simulink model "w3_warplab_buffers"  (Simulink 7.7)
settings: Solver=VariableStepDiscrete  SolverMode=SingleTasking  StartTime=0.0  StopTime=200000  RelTol=1e-3
InitFcn:
  | w3_warplab_buffers_init
StartFcn:
  | w3_warplab_buffers_init
values from neighbouring files (symbols this model uses):
  NumSamps_Rx_IQ = 2^15    (= 32768)    [w3_warplab_buffers_init.m]
  NumSamps_Rx_RSSI = 2^13    (= 8192)    [w3_warplab_buffers_init.m]
  NumSamps_Tx_IQ = 2^15    (= 32768)    [w3_warplab_buffers_init.m]
undefined symbols (not defined in the file or in its folder): gcbh, xlBlockLoadCallback, xlGetNormalizedPeriod
libraries: xbsIndex_r4 x1266, xbsEDKLib_r4 x1
(part 3 of 9)

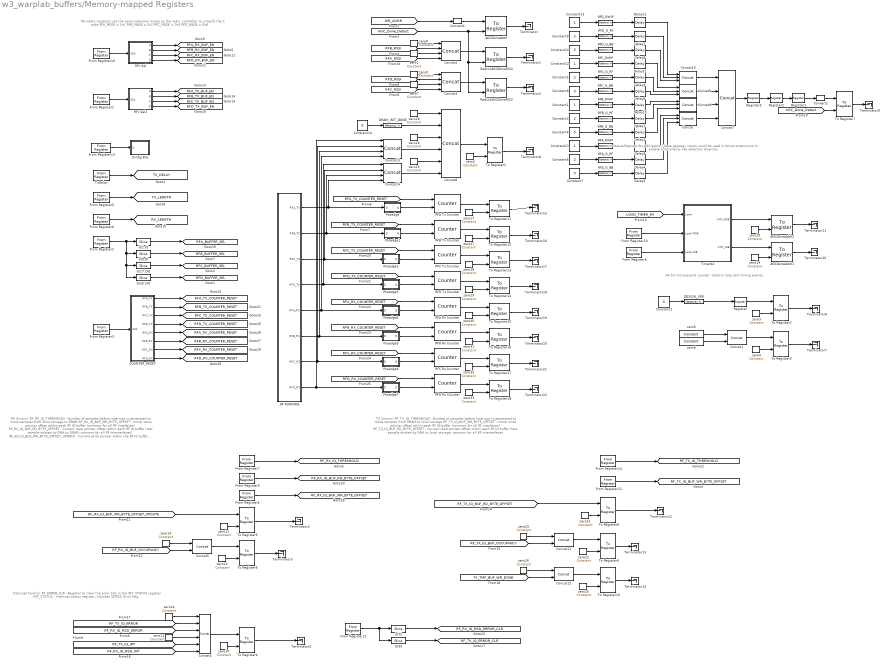
== system w3_warplab_buffers/Memory-mapped Registers ==
  note: Per-radio registers use the same selection
      | masks as the radio_controller to simplify the C code
      | RFA_MASK = 0x1
      | RFB_MASK = 0x2
      | RFC_MASK = 0x4
      | RFD_MASK = 0x8
  note: RX Control:
      |     RF_RX_IQ_THRESHOLD                                      - Number of samples before interrupt is generated to move samples from local storage to DRAM
      |     RF_RX_IQ_BUF_WR_BYTE_OFFSET                  - Initial write pointer offset within each RF IQ buffer (common for all RF interfaces)
      |     RF_RX_IQ_BUF_RD_BYTE_OFFSET                   - Current read pointer offset within each RF IQ buffer (last sample written by DMA to DRAM; common for all RF interterfaces)
      |     RF_RX_IQ_BUF_WR_BYTE_OFFSET_UPDATE  - Current write pointer within the RF IQ buffer (last sample written by RF interface; common for all RF interfaces)
  note: Status Register for AGC gains.  These gateway inputs could be used in future extensions to
      | enable functionality like selection diveristy.
  note: 64 bit microsecond counter. Used to help with timing events.
  note: TX Control:
      |     RF_TX_IQ_THRESHOLD                                      - Number of samples before interrupt is generated to move samples from DRAM to local storage
      |     RF_TX_IQ_BUF_WR_BYTE_OFFSET                  - Initial write pointer offset within each RF IQ buffer (common for all RF interfaces)
      |     RF_TX_IQ_BUF_RD_BYTE_OFFSET                   - Current read pointer offset within each RF IQ buffer (last sample written by DMA to local storage; common for all RF interterfaces
  note: Interrupt Control:
      |     RF_ERROR_CLR                                                   - Register to clear the error bits in the INT_STATUS register
      |     INT_STATUS                                                        - Interrupt status register; Includes IQ/RSSI Error flag
  AGCDoneAddr : xbsIndex_r4/To Register  shared_memory_name='AGC_DONE_ADDR'  init=0  ownership=Locally owned and initialized  explicit_data_type=on  gui_display_data_type=Fixed-point  arith_type=Unsigned  n_bits=32  bin_pt=0  preci_type=Single  dbl_ovrd=off  block_type=toreg
      settings: AttributesFormatString=<< %<shared_memory_name> >>  infoedit="Register block that writes data to a shared memory register.  Delay of one sample period."  block_version=10.1.3
  AGCDoneAddr1 : xbsIndex_r4/To Register  shared_memory_name='TIMER_64_LSB'  init=0  ownership=Locally owned and initialized  explicit_data_type=on  gui_display_data_type=Fixed-point  arith_type=Unsigned  n_bits=32  bin_pt=0  preci_type=Single  dbl_ovrd=off  block_type=toreg
      settings: AttributesFormatString=<< %<shared_memory_name> >>  infoedit="Register block that writes data to a shared memory register.  Delay of one sample period."  block_version=10.1.3
  AGCDoneAddr2 : xbsIndex_r4/To Register  shared_memory_name='TIMER_64_MSB'  init=0  ownership=Locally owned and initialized  explicit_data_type=on  gui_display_data_type=Fixed-point  arith_type=Unsigned  n_bits=32  bin_pt=0  preci_type=Single  dbl_ovrd=off  block_type=toreg
      settings: AttributesFormatString=<< %<shared_memory_name> >>  infoedit="Register block that writes data to a shared memory register.  Delay of one sample period."  block_version=10.1.3
  COUNTER_RESET : Subsystem
  Concat{,8..10} (4 alike) : xbsIndex_r4/Concat  num_inputs=3  dbl_ovrd=off  block_type=concat
  Concat{1,5,11..12} (4 alike) : xbsIndex_r4/Concat  num_inputs=2  dbl_ovrd=off  block_type=concat
  Concat{2..3,7,13..14} (5 alike) : xbsIndex_r4/Concat  num_inputs=4  dbl_ovrd=off  block_type=concat
  Concat4 : xbsIndex_r4/Concat  num_inputs=6  dbl_ovrd=off  block_type=concat
  Concat6 : xbsIndex_r4/Concat  num_inputs=6  dbl_ovrd=off  block_type=concat
  Config Bits : Subsystem
  Constant{1,11..13} (4 alike) : Constant
  Constant{4,7..8,10} (4 alike) : Constant  Value=5
  Constant14 : Constant  Value=0
  Constant2 : Constant  Value=0
  Constant{3,5..6,9} (4 alike) : Constant  Value=2
  Convert1 : xbsIndex_r4/Convert  gui_display_data_type=Fixed-point  arith_type=Unsigned  n_bits=32  bin_pt=0  float_type=Single  exp_bits=8  fraction_bits=24  quantization=Truncate  overflow=Wrap  en=off  latency=0  dbl_ovrd=off  pipeline=off  block_type=convert
      settings: block_version=8.2
  Convert4 : xbsIndex_r4/Convert  gui_display_data_type=Fixed-point  arith_type=Unsigned  n_bits=32  bin_pt=0  float_type=Single  exp_bits=8  fraction_bits=24  quantization=Truncate  overflow=Wrap  en=off  latency=0  dbl_ovrd=off  pipeline=off  block_type=convert
      settings: block_version=8.2
  DESIGN_VER : xbsIndex_r4/Gateway In  gui_display_data_type=Fixed-point  arith_type=Unsigned  n_bits=32  bin_pt=0  preci_type=Single  exp_width=8  frac_width=24  quantization="Round  (unbiased: +/- Inf)"  overflow=Saturate  period=1  dbl_ovrd=off  timing_constraint=None  locs_specified=off  LOCs={}  UseAsADC=off  ADCChannel='1'  inherit_from_input=off  hdl_port=on  block_type=gatewayin
      settings: block_version=VER_STRING_GOES_HERE
  DRAM_INIT_DONE : xbsIndex_r4/Gateway In  gui_display_data_type=Fixed-point  arith_type=Unsigned  n_bits=1  bin_pt=0  preci_type=Single  exp_width=8  frac_width=24  quantization="Round  (unbiased: +/- Inf)"  overflow=Saturate  period=1  dbl_ovrd=off  timing_constraint=None  locs_specified=off  LOCs={}  UseAsADC=off  ADCChannel='1'  inherit_from_input=off  hdl_port=on  block_type=gatewayin
      settings: block_version=VER_STRING_GOES_HERE
  Delay{1..12} (12 alike) : xbsIndex_r4/Delay  rst=off  infoeditControl=Selection of Reset will increase slice count due to use of real FFs and instead of SRLs  en=off  latency=1  dbl_ovrd=off  reg_retiming=off  block_type=delay
  From Register1 : xbsIndex_r4/From Register  shared_memory_name='TX_BUF_EN'  init=tx_buf_en  period=1  ownership=Locally owned and initialized  gui_display_data_type=Fixed-point  arith_type=Unsigned  n_bits=32  bin_pt=0  preci_type=Single  dbl_ovrd=off  block_type=fromreg
      settings: AttributesFormatString=<< %<shared_memory_name> >>  infoedit="Register block that reads data to a shared memory register.  Delay of one sample period."  block_version=8.2
  From Register10 : xbsIndex_r4/From Register  shared_memory_name='LOAD_TIMER_64_MSB'  init=0  period=1  ownership=Locally owned and initialized  gui_display_data_type=Fixed-point  arith_type=Unsigned  n_bits=32  bin_pt=0  preci_type=Single  dbl_ovrd=off  block_type=fromreg
      settings: AttributesFormatString=<< %<shared_memory_name> >>  infoedit="Register block that reads data to a shared memory register.  Delay of one sample period."  block_version=8.2
  From Register11 : xbsIndex_r4/From Register  shared_memory_name='RF_TX_IQ_BUF_WR_BYTE_OFFSET'  init=rf_tx_iq_buf_wr_byte_offset  period=1  ownership=Locally owned and initialized  gui_display_data_type=Fixed-point  arith_type=Unsigned  n_bits=32  bin_pt=0  preci_type=Single  dbl_ovrd=off  block_type=fromreg
      settings: AttributesFormatString=<< %<shared_memory_name> >>  infoedit="Register block that reads data to a shared memory register.  Delay of one sample period."  block_version=8.2
  From Register12 : xbsIndex_r4/From Register  shared_memory_name='RF_ERROR_CLR'  init=rf_error_clr  period=1  ownership=Locally owned and initialized  gui_display_data_type=Fixed-point  arith_type=Unsigned  n_bits=9  bin_pt=0  preci_type=Single  dbl_ovrd=off  block_type=fromreg
      settings: AttributesFormatString=<< %<shared_memory_name> >>  infoedit="Register block that reads data to a shared memory register.  Delay of one sample period."  block_version=8.2
  From Register13 : xbsIndex_r4/From Register  shared_memory_name='CONFIG'  init=wl_buffers_config_init  period=1  ownership=Locally owned and initialized  gui_display_data_type=Fixed-point  arith_type=Unsigned  n_bits=32  bin_pt=0  preci_type=Single  dbl_ovrd=off  block_type=fromreg
      settings: AttributesFormatString=<< %<shared_memory_name> >>  infoedit="Register block that reads data to a shared memory register.  Delay of one sample period."
  From Register14 : xbsIndex_r4/From Register  shared_memory_name='RF_TX_IQ_THRESHOLD'  init=rf_tx_iq_threshold  period=1  ownership=Locally owned and initialized  gui_display_data_type=Fixed-point  arith_type=Unsigned  n_bits=32  bin_pt=0  preci_type=Single  dbl_ovrd=off  block_type=fromreg
      settings: AttributesFormatString=<< %<shared_memory_name> >>  infoedit="Register block that reads data to a shared memory register.  Delay of one sample period."  block_version=8.2
  From Register16 : xbsIndex_r4/From Register  shared_memory_name='RX_BUF_EN'  init=rx_buf_en  period=1  ownership=Locally owned and initialized  gui_display_data_type=Fixed-point  arith_type=Unsigned  n_bits=32  bin_pt=0  preci_type=Single  dbl_ovrd=off  block_type=fromreg
      settings: AttributesFormatString=<< %<shared_memory_name> >>  infoedit="Register block that reads data to a shared memory register.  Delay of one sample period."  block_version=8.2
  From Register2 : xbsIndex_r4/From Register  shared_memory_name='RF_BUFFER_SEL'  init=wl_buffers_rf_buffer_sel  period=1  ownership=Locally owned and initialized  gui_display_data_type=Fixed-point  arith_type=Unsigned  n_bits=32  bin_pt=0  preci_type=Single  dbl_ovrd=off  block_type=fromreg
      settings: AttributesFormatString=<< %<shared_memory_name> >>  infoedit="Register block that reads data to a shared memory register.  Delay of one sample period."  block_version=8.2
  From Register3 : xbsIndex_r4/From Register  shared_memory_name='TXRX_COUNTER_RESET'  init=txrx_counter_reset  period=1  ownership=Locally owned and initialized  gui_display_data_type=Fixed-point  arith_type=Unsigned  n_bits=32  bin_pt=0  preci_type=Single  dbl_ovrd=off  block_type=fromreg
      settings: AttributesFormatString=<< %<shared_memory_name> >>  infoedit="Register block that reads data to a shared memory register.  Delay of one sample period."  block_version=8.2
  From Register4 : xbsIndex_r4/From Register  shared_memory_name='RF_RX_IQ_BUF_WR_BYTE_OFFSET'  init=rf_rx_iq_buf_wr_byte_offset  period=1  ownership=Locally owned and initialized  gui_display_data_type=Fixed-point  arith_type=Unsigned  n_bits=32  bin_pt=0  preci_type=Single  dbl_ovrd=off  block_type=fromreg
      settings: AttributesFormatString=<< %<shared_memory_name> >>  infoedit="Register block that reads data to a shared memory register.  Delay of one sample period."  block_version=8.2
  From Register5 : xbsIndex_r4/From Register  shared_memory_name='TX_LENGTH'  init=tx_length  period=1  ownership=Locally owned and initialized  gui_display_data_type=Fixed-point  arith_type=Unsigned  n_bits=32  bin_pt=0  preci_type=Single  dbl_ovrd=off  block_type=fromreg
      settings: AttributesFormatString=<< %<shared_memory_name> >>  infoedit="Register block that reads data to a shared memory register.  Delay of one sample period."  block_version=8.2
  From Register6 : xbsIndex_r4/From Register  shared_memory_name='RX_LENGTH'  init=rx_length  period=1  ownership=Locally owned and initialized  gui_display_data_type=Fixed-point  arith_type=Unsigned  n_bits=32  bin_pt=0  preci_type=Single  dbl_ovrd=off  block_type=fromreg
      settings: AttributesFormatString=<< %<shared_memory_name> >>  infoedit="Register block that reads data to a shared memory register.  Delay of one sample period."  block_version=8.2
  From Register7 : xbsIndex_r4/From Register  shared_memory_name='RF_RX_IQ_THRESHOLD'  init=rf_rx_iq_threshold  period=1  ownership=Locally owned and initialized  gui_display_data_type=Fixed-point  arith_type=Unsigned  n_bits=32  bin_pt=0  preci_type=Single  dbl_ovrd=off  block_type=fromreg
      settings: AttributesFormatString=<< %<shared_memory_name> >>  infoedit="Register block that reads data to a shared memory register.  Delay of one sample period."  block_version=8.2
  From Register8 : xbsIndex_r4/From Register  shared_memory_name='LOAD_TIMER_64_LSB'  init=0  period=1  ownership=Locally owned and initialized  gui_display_data_type=Fixed-point  arith_type=Unsigned  n_bits=32  bin_pt=0  preci_type=Single  dbl_ovrd=off  block_type=fromreg
      settings: AttributesFormatString=<< %<shared_memory_name> >>  infoedit="Register block that reads data to a shared memory register.  Delay of one sample period."  block_version=8.2
  From Register9 : xbsIndex_r4/From Register  shared_memory_name='RF_RX_IQ_BUF_RD_BYTE_OFFSET'  init=rf_rx_iq_buf_rd_byte_offset  period=1  ownership=Locally owned and initialized  gui_display_data_type=Fixed-point  arith_type=Unsigned  n_bits=32  bin_pt=0  preci_type=Single  dbl_ovrd=off  block_type=fromreg
      settings: AttributesFormatString=<< %<shared_memory_name> >>  infoedit="Register block that reads data to a shared memory register.  Delay of one sample period."  block_version=8.2
  Posedge : Subsystem
  Posedge1 : Subsystem
  Posedge2 : Subsystem
  Posedge3 : Subsystem
  Posedge4 : Subsystem
  Posedge5 : Subsystem
  Posedge6 : Subsystem
  Posedge7 : Subsystem
  RF RUNNING : Subsystem
  RFA Rx Counter : xbsIndex_r4/Counter  cnt_type=Free Running  cnt_to=Inf  operation=Up  start_count=0  cnt_by_val=1  arith_type=Unsigned  n_bits=32  bin_pt=0  load_pin=off  rst=on  en=on  explicit_period=off  period=1  dbl_ovrd=off  use_behavioral_HDL=off  implementation=Fabric  use_rpm=off  block_type=counter
      settings: block_version=8.2
  RFA Tx Counter : xbsIndex_r4/Counter  cnt_type=Free Running  cnt_to=Inf  operation=Up  start_count=0  cnt_by_val=1  arith_type=Unsigned  n_bits=32  bin_pt=0  load_pin=off  rst=on  en=on  explicit_period=off  period=1  dbl_ovrd=off  use_behavioral_HDL=off  implementation=Fabric  use_rpm=off  block_type=counter
      settings: block_version=8.2
  RFA_G_BB : xbsIndex_r4/Gateway In  gui_display_data_type=Fixed-point  arith_type=Unsigned  n_bits=5  bin_pt=0  preci_type=Single  exp_width=8  frac_width=24  quantization="Round  (unbiased: +/- Inf)"  overflow=Saturate  period=1  dbl_ovrd=off  timing_constraint=None  locs_specified=off  LOCs={}  UseAsADC=off  ADCChannel='1'  inherit_from_input=off  hdl_port=on  block_type=gatewayin
  RFA_G_RF : xbsIndex_r4/Gateway In  gui_display_data_type=Fixed-point  arith_type=Unsigned  n_bits=2  bin_pt=0  preci_type=Single  exp_width=8  frac_width=24  quantization="Round  (unbiased: +/- Inf)"  overflow=Saturate  period=1  dbl_ovrd=off  timing_constraint=None  locs_specified=off  LOCs={}  UseAsADC=off  ADCChannel='1'  inherit_from_input=off  hdl_port=on  block_type=gatewayin
  RFA_RXHP : xbsIndex_r4/Gateway In  gui_display_data_type=Fixed-point  arith_type=Unsigned  n_bits=1  bin_pt=0  preci_type=Single  exp_width=8  frac_width=24  quantization="Round  (unbiased: +/- Inf)"  overflow=Saturate  period=1  dbl_ovrd=off  timing_constraint=None  locs_specified=off  LOCs={}  UseAsADC=off  ADCChannel='1'  inherit_from_input=off  hdl_port=on  block_type=gatewayin
  RFB Rx Counter : xbsIndex_r4/Counter  cnt_type=Free Running  cnt_to=Inf  operation=Up  start_count=0  cnt_by_val=1  arith_type=Unsigned  n_bits=32  bin_pt=0  load_pin=off  rst=on  en=on  explicit_period=off  period=1  dbl_ovrd=off  use_behavioral_HDL=off  implementation=Fabric  use_rpm=off  block_type=counter
      settings: block_version=8.2
  RFB Tx Counter : xbsIndex_r4/Counter  cnt_type=Free Running  cnt_to=Inf  operation=Up  start_count=0  cnt_by_val=1  arith_type=Unsigned  n_bits=32  bin_pt=0  load_pin=off  rst=on  en=on  explicit_period=off  period=1  dbl_ovrd=off  use_behavioral_HDL=off  implementation=Fabric  use_rpm=off  block_type=counter
      settings: block_version=8.2
  RFB_G_BB : xbsIndex_r4/Gateway In  gui_display_data_type=Fixed-point  arith_type=Unsigned  n_bits=5  bin_pt=0  preci_type=Single  exp_width=8  frac_width=24  quantization="Round  (unbiased: +/- Inf)"  overflow=Saturate  period=1  dbl_ovrd=off  timing_constraint=None  locs_specified=off  LOCs={}  UseAsADC=off  ADCChannel='1'  inherit_from_input=off  hdl_port=on  block_type=gatewayin
  RFB_G_RF : xbsIndex_r4/Gateway In  gui_display_data_type=Fixed-point  arith_type=Unsigned  n_bits=2  bin_pt=0  preci_type=Single  exp_width=8  frac_width=24  quantization="Round  (unbiased: +/- Inf)"  overflow=Saturate  period=1  dbl_ovrd=off  timing_constraint=None  locs_specified=off  LOCs={}  UseAsADC=off  ADCChannel='1'  inherit_from_input=off  hdl_port=on  block_type=gatewayin
  RFB_RXHP : xbsIndex_r4/Gateway In  gui_display_data_type=Fixed-point  arith_type=Unsigned  n_bits=1  bin_pt=0  preci_type=Single  exp_width=8  frac_width=24  quantization="Round  (unbiased: +/- Inf)"  overflow=Saturate  period=1  dbl_ovrd=off  timing_constraint=None  locs_specified=off  LOCs={}  UseAsADC=off  ADCChannel='1'  inherit_from_input=off  hdl_port=on  block_type=gatewayin
  RFC Rx Counter : xbsIndex_r4/Counter  cnt_type=Free Running  cnt_to=Inf  operation=Up  start_count=0  cnt_by_val=1  arith_type=Unsigned  n_bits=32  bin_pt=0  load_pin=off  rst=on  en=on  explicit_period=off  period=1  dbl_ovrd=off  use_behavioral_HDL=off  implementation=Fabric  use_rpm=off  block_type=counter
      settings: block_version=8.2
  RFC Tx Counter : xbsIndex_r4/Counter  cnt_type=Free Running  cnt_to=Inf  operation=Up  start_count=0  cnt_by_val=1  arith_type=Unsigned  n_bits=32  bin_pt=0  load_pin=off  rst=on  en=on  explicit_period=off  period=1  dbl_ovrd=off  use_behavioral_HDL=off  implementation=Fabric  use_rpm=off  block_type=counter
      settings: block_version=8.2
  RFC_G_BB : xbsIndex_r4/Gateway In  gui_display_data_type=Fixed-point  arith_type=Unsigned  n_bits=5  bin_pt=0  preci_type=Single  exp_width=8  frac_width=24  quantization="Round  (unbiased: +/- Inf)"  overflow=Saturate  period=1  dbl_ovrd=off  timing_constraint=None  locs_specified=off  LOCs={}  UseAsADC=off  ADCChannel='1'  inherit_from_input=off  hdl_port=on  block_type=gatewayin
  RFC_G_RF : xbsIndex_r4/Gateway In  gui_display_data_type=Fixed-point  arith_type=Unsigned  n_bits=2  bin_pt=0  preci_type=Single  exp_width=8  frac_width=24  quantization="Round  (unbiased: +/- Inf)"  overflow=Saturate  period=1  dbl_ovrd=off  timing_constraint=None  locs_specified=off  LOCs={}  UseAsADC=off  ADCChannel='1'  inherit_from_input=off  hdl_port=on  block_type=gatewayin
  RFC_RXHP : xbsIndex_r4/Gateway In  gui_display_data_type=Fixed-point  arith_type=Unsigned  n_bits=1  bin_pt=0  preci_type=Single  exp_width=8  frac_width=24  quantization="Round  (unbiased: +/- Inf)"  overflow=Saturate  period=1  dbl_ovrd=off  timing_constraint=None  locs_specified=off  LOCs={}  UseAsADC=off  ADCChannel='1'  inherit_from_input=off  hdl_port=on  block_type=gatewayin
  RFD Rx Counter : xbsIndex_r4/Counter  cnt_type=Free Running  cnt_to=Inf  operation=Up  start_count=0  cnt_by_val=1  arith_type=Unsigned  n_bits=32  bin_pt=0  load_pin=off  rst=on  en=on  explicit_period=off  period=1  dbl_ovrd=off  use_behavioral_HDL=off  implementation=Fabric  use_rpm=off  block_type=counter
      settings: block_version=8.2
  RFD Tx Counter : xbsIndex_r4/Counter  cnt_type=Free Running  cnt_to=Inf  operation=Up  start_count=0  cnt_by_val=1  arith_type=Unsigned  n_bits=32  bin_pt=0  load_pin=off  rst=on  en=on  explicit_period=off  period=1  dbl_ovrd=off  use_behavioral_HDL=off  implementation=Fabric  use_rpm=off  block_type=counter
      settings: block_version=8.2
  RFD_G_BB : xbsIndex_r4/Gateway In  gui_display_data_type=Fixed-point  arith_type=Unsigned  n_bits=5  bin_pt=0  preci_type=Single  exp_width=8  frac_width=24  quantization="Round  (unbiased: +/- Inf)"  overflow=Saturate  period=1  dbl_ovrd=off  timing_constraint=None  locs_specified=off  LOCs={}  UseAsADC=off  ADCChannel='1'  inherit_from_input=off  hdl_port=on  block_type=gatewayin
  RFD_G_RF : xbsIndex_r4/Gateway In  gui_display_data_type=Fixed-point  arith_type=Unsigned  n_bits=2  bin_pt=0  preci_type=Single  exp_width=8  frac_width=24  quantization="Round  (unbiased: +/- Inf)"  overflow=Saturate  period=1  dbl_ovrd=off  timing_constraint=None  locs_specified=off  LOCs={}  UseAsADC=off  ADCChannel='1'  inherit_from_input=off  hdl_port=on  block_type=gatewayin
  RFD_RXHP : xbsIndex_r4/Gateway In  gui_display_data_type=Fixed-point  arith_type=Unsigned  n_bits=1  bin_pt=0  preci_type=Single  exp_width=8  frac_width=24  quantization="Round  (unbiased: +/- Inf)"  overflow=Saturate  period=1  dbl_ovrd=off  timing_constraint=None  locs_specified=off  LOCs={}  UseAsADC=off  ADCChannel='1'  inherit_from_input=off  hdl_port=on  block_type=gatewayin
  RFx Sel : Subsystem
  RFx Sel2 : Subsystem
  Radio1AGCDoneRSSI : xbsIndex_r4/To Register  shared_memory_name='RFAB_AGC_DONE_RSSI'  init=0  ownership=Locally owned and initialized  explicit_data_type=on  gui_display_data_type=Fixed-point  arith_type=Unsigned  n_bits=32  bin_pt=0  preci_type=Single  dbl_ovrd=off  block_type=toreg
      settings: AttributesFormatString=<< %<shared_memory_name> >>  infoedit="Register block that writes data to a shared memory register.  Delay of one sample period."  block_version=10.1.3
  Radio3AGCDoneRSSI : xbsIndex_r4/To Register  shared_memory_name='RFCD_AGC_DONE_RSSI'  init=0  ownership=Locally owned and initialized  explicit_data_type=on  gui_display_data_type=Fixed-point  arith_type=Unsigned  n_bits=32  bin_pt=0  preci_type=Single  dbl_ovrd=off  block_type=toreg
      settings: AttributesFormatString=<< %<shared_memory_name> >>  infoedit="Register block that writes data to a shared memory register.  Delay of one sample period."  block_version=10.1.3
  Register{,1..3} (4 alike) : xbsIndex_r4/Register  init=0  rst=off  en=off  dbl_ovrd=off  block_type=register
      settings: block_version=8.2
  Terminator{,1..22} (23 alike) : Terminator
  Timer64 : Subsystem
  To Register1 : xbsIndex_r4/To Register  shared_memory_name='STATUS'  init=0  ownership=Locally owned and initialized  explicit_data_type=on  gui_display_data_type=Fixed-point  arith_type=Unsigned  n_bits=32  bin_pt=0  preci_type=Single  dbl_ovrd=off  block_type=toreg
      settings: AttributesFormatString=<< %<shared_memory_name> >>  infoedit="Register block that writes data to a shared memory register.  Delay of one sample period."  block_version=8.2
  To Register10 : xbsIndex_r4/To Register  shared_memory_name='RF_TX_IQ_STATUS'  init=0  ownership=Locally owned and initialized  explicit_data_type=on  gui_display_data_type=Fixed-point  arith_type=Unsigned  n_bits=32  bin_pt=0  preci_type=Single  dbl_ovrd=off  block_type=toreg
      settings: AttributesFormatString=<< %<shared_memory_name> >>  infoedit="Register block that writes data to a shared memory register.  Delay of one sample period."  block_version=8.2
  To Register11 : xbsIndex_r4/To Register  shared_memory_name='RFA_TX_COUNTER'  init=0  ownership=Locally owned and initialized  explicit_data_type=on  gui_display_data_type=Fixed-point  arith_type=Unsigned  n_bits=32  bin_pt=0  preci_type=Single  dbl_ovrd=off  block_type=toreg
      settings: AttributesFormatString=<< %<shared_memory_name> >>  infoedit="Register block that writes data to a shared memory register.  Delay of one sample period."  block_version=8.2
  To Register12 : xbsIndex_r4/To Register  shared_memory_name='RFB_TX_COUNTER'  init=0  ownership=Locally owned and initialized  explicit_data_type=on  gui_display_data_type=Fixed-point  arith_type=Unsigned  n_bits=32  bin_pt=0  preci_type=Single  dbl_ovrd=off  block_type=toreg
      settings: AttributesFormatString=<< %<shared_memory_name> >>  infoedit="Register block that writes data to a shared memory register.  Delay of one sample period."  block_version=8.2
  To Register13 : xbsIndex_r4/To Register  shared_memory_name='RFC_TX_COUNTER'  init=0  ownership=Locally owned and initialized  explicit_data_type=on  gui_display_data_type=Fixed-point  arith_type=Unsigned  n_bits=32  bin_pt=0  preci_type=Single  dbl_ovrd=off  block_type=toreg
      settings: AttributesFormatString=<< %<shared_memory_name> >>  infoedit="Register block that writes data to a shared memory register.  Delay of one sample period."  block_version=8.2
  To Register14 : xbsIndex_r4/To Register  shared_memory_name='RFD_TX_COUNTER'  init=0  ownership=Locally owned and initialized  explicit_data_type=on  gui_display_data_type=Fixed-point  arith_type=Unsigned  n_bits=32  bin_pt=0  preci_type=Single  dbl_ovrd=off  block_type=toreg
      settings: AttributesFormatString=<< %<shared_memory_name> >>  infoedit="Register block that writes data to a shared memory register.  Delay of one sample period."  block_version=8.2
  To Register15 : xbsIndex_r4/To Register  shared_memory_name='RFA_RX_COUNTER'  init=0  ownership=Locally owned and initialized  explicit_data_type=on  gui_display_data_type=Fixed-point  arith_type=Unsigned  n_bits=32  bin_pt=0  preci_type=Single  dbl_ovrd=off  block_type=toreg
      settings: AttributesFormatString=<< %<shared_memory_name> >>  infoedit="Register block that writes data to a shared memory register.  Delay of one sample period."  block_version=8.2
  To Register16 : xbsIndex_r4/To Register  shared_memory_name='RFB_RX_COUNTER'  init=0  ownership=Locally owned and initialized  explicit_data_type=on  gui_display_data_type=Fixed-point  arith_type=Unsigned  n_bits=32  bin_pt=0  preci_type=Single  dbl_ovrd=off  block_type=toreg
      settings: AttributesFormatString=<< %<shared_memory_name> >>  infoedit="Register block that writes data to a shared memory register.  Delay of one sample period."  block_version=8.2
  To Register17 : xbsIndex_r4/To Register  shared_memory_name='RFC_RX_COUNTER'  init=0  ownership=Locally owned and initialized  explicit_data_type=on  gui_display_data_type=Fixed-point  arith_type=Unsigned  n_bits=32  bin_pt=0  preci_type=Single  dbl_ovrd=off  block_type=toreg
      settings: AttributesFormatString=<< %<shared_memory_name> >>  infoedit="Register block that writes data to a shared memory register.  Delay of one sample period."  block_version=8.2
  To Register18 : xbsIndex_r4/To Register  shared_memory_name='RFD_RX_COUNTER'  init=0  ownership=Locally owned and initialized  explicit_data_type=on  gui_display_data_type=Fixed-point  arith_type=Unsigned  n_bits=32  bin_pt=0  preci_type=Single  dbl_ovrd=off  block_type=toreg
      settings: AttributesFormatString=<< %<shared_memory_name> >>  infoedit="Register block that writes data to a shared memory register.  Delay of one sample period."  block_version=8.2
  To Register2 : xbsIndex_r4/To Register  shared_memory_name='DESIGN_VER'  init=0  ownership=Locally owned and initialized  explicit_data_type=on  gui_display_data_type=Fixed-point  arith_type=Unsigned  n_bits=32  bin_pt=0  preci_type=Single  dbl_ovrd=off  block_type=toreg
      settings: AttributesFormatString=<< %<shared_memory_name> >>  infoedit="Register block that writes data to a shared memory register.  Delay of one sample period."  block_version=8.2
  To Register3 : xbsIndex_r4/To Register  shared_memory_name='BUFF_SIZES'  init=0  ownership=Locally owned and initialized  explicit_data_type=on  gui_display_data_type=Fixed-point  arith_type=Unsigned  n_bits=32  bin_pt=0  preci_type=Single  dbl_ovrd=off  block_type=toreg
      settings: AttributesFormatString=<< %<shared_memory_name> >>  infoedit="Register block that writes data to a shared memory register.  Delay of one sample period."  block_version=8.2
  To Register4 : xbsIndex_r4/To Register  shared_memory_name='INT_STATUS'  init=0  ownership=Locally owned and initialized  explicit_data_type=on  gui_display_data_type=Fixed-point  arith_type=Unsigned  n_bits=32  bin_pt=0  preci_type=Single  dbl_ovrd=off  block_type=toreg
      settings: AttributesFormatString=<< %<shared_memory_name> >>  infoedit="Register block that writes data to a shared memory register.  Delay of one sample period."  block_version=8.2
  To Register5 : xbsIndex_r4/To Register  shared_memory_name='RF_RX_IQ_BUF_WR_BYTE_OFFSET_UPDATE'  init=0  ownership=Locally owned and initialized  explicit_data_type=on  gui_display_data_type=Fixed-point  arith_type=Unsigned  n_bits=32  bin_pt=0  preci_type=Single  dbl_ovrd=off  block_type=toreg
      settings: AttributesFormatString=<< %<shared_memory_name> >>  infoedit="Register block that writes data to a shared memory register.  Delay of one sample period."  block_version=8.2
  To Register6 : xbsIndex_r4/To Register  shared_memory_name='RF_RX_IQ_BUF_OCCUPANCY'  init=0  ownership=Locally owned and initialized  explicit_data_type=on  gui_display_data_type=Fixed-point  arith_type=Unsigned  n_bits=32  bin_pt=0  preci_type=Single  dbl_ovrd=off  block_type=toreg
      settings: AttributesFormatString=<< %<shared_memory_name> >>  infoedit="Register block that writes data to a shared memory register.  Delay of one sample period."  block_version=8.2
  To Register7 : xbsIndex_r4/To Register  shared_memory_name='AGC_GAINS'  init=0  ownership=Locally owned and initialized  explicit_data_type=on  gui_display_data_type=Fixed-point  arith_type=Unsigned  n_bits=32  bin_pt=0  preci_type=Single  dbl_ovrd=off  block_type=toreg
      settings: AttributesFormatString=<< %<shared_memory_name> >>  infoedit="Register block that writes data to a shared memory register.  Delay of one sample period."  block_version=8.2
  To Register8 : xbsIndex_r4/To Register  shared_memory_name='RF_TX_IQ_BUF_RD_BYTE_OFFSET'  init=0  ownership=Locally owned and initialized  explicit_data_type=on  gui_display_data_type=Fixed-point  arith_type=Unsigned  n_bits=32  bin_pt=0  preci_type=Single  dbl_ovrd=off  block_type=toreg
      settings: AttributesFormatString=<< %<shared_memory_name> >>  infoedit="Register block that writes data to a shared memory register.  Delay of one sample period."  block_version=8.2
  To Register9 : xbsIndex_r4/To Register  shared_memory_name='RF_TX_IQ_BUF_OCCUPANCY'  init=0  ownership=Locally owned and initialized  explicit_data_type=on  gui_display_data_type=Fixed-point  arith_type=Unsigned  n_bits=32  bin_pt=0  preci_type=Single  dbl_ovrd=off  block_type=toreg
      settings: AttributesFormatString=<< %<shared_memory_name> >>  infoedit="Register block that writes data to a shared memory register.  Delay of one sample period."  block_version=8.2
  TxDelay : xbsIndex_r4/From Register  shared_memory_name='TX_DELAY'  init=wl_buffers_tx_delay_init  period=1  ownership=Locally owned and initialized  gui_display_data_type=Fixed-point  arith_type=Unsigned  n_bits=32  bin_pt=0  preci_type=Single  dbl_ovrd=off  block_type=fromreg
      settings: AttributesFormatString=<< %<shared_memory_name> >>  infoedit="Register block that reads data to a shared memory register.  Delay of one sample period."  block_version=10.1.2
  b[0] : xbsIndex_r4/Slice  nbits=1  boolean_output=off  mode=Lower Bit Location + Width  bit1=0  base1=MSB of Input  bit0=0  base0=LSB of Input  dbl_ovrd=off  block_type=slice
  b[17:16] : xbsIndex_r4/Slice  nbits=2  boolean_output=off  mode=Lower Bit Location + Width  bit1=0  base1=MSB of Input  bit0=16  base0=LSB of Input  dbl_ovrd=off  block_type=slice
  b[1:0] : xbsIndex_r4/Slice  nbits=2  boolean_output=off  mode=Lower Bit Location + Width  bit1=0  base1=MSB of Input  bit0=0  base0=LSB of Input  dbl_ovrd=off  block_type=slice
  b[25:24] : xbsIndex_r4/Slice  nbits=2  boolean_output=off  mode=Lower Bit Location + Width  bit1=0  base1=MSB of Input  bit0=24  base0=LSB of Input  dbl_ovrd=off  block_type=slice
  b[8] : xbsIndex_r4/Slice  nbits=1  boolean_output=off  mode=Lower Bit Location + Width  bit1=0  base1=MSB of Input  bit0=8  base0=LSB of Input  dbl_ovrd=off  block_type=slice
  b[9:8] : xbsIndex_r4/Slice  nbits=2  boolean_output=off  mode=Lower Bit Location + Width  bit1=0  base1=MSB of Input  bit0=8  base0=LSB of Input  dbl_ovrd=off  block_type=slice
  zero{1,7..9,24} (5 alike) : xbsIndex_r4/Constant  const=0  gui_display_data_type=Fixed-point  arith_type=Unsigned  n_bits=6  bin_pt=0  preci_type=Single  exp_width=8  frac_width=24  explicit_period=off  period=1  equ=P=C  opselect=C  inp2=PCIN>>17  opr=+  inp1=P  carry=CIN  dbl_ovrd=off  block_type=constant
      settings: block_version=VER_STRING_GOES_HERE
  zero{2..4,10,12..13,17,19..22,25,27..33} (19 alike) : xbsIndex_r4/Constant  const=1  gui_display_data_type=Fixed-point  arith_type=Boolean  n_bits=1  bin_pt=0  preci_type=Single  exp_width=8  frac_width=24  explicit_period=off  period=1  equ=P=C  opselect=C  inp2=PCIN>>17  opr=+  inp1=P  carry=CIN  dbl_ovrd=off  block_type=constant
      settings: block_version=VER_STRING_GOES_HERE
  zero11 : xbsIndex_r4/Constant  const=0  gui_display_data_type=Fixed-point  arith_type=Unsigned  n_bits=22  bin_pt=0  preci_type=Single  exp_width=8  frac_width=24  explicit_period=off  period=1  equ=P=C  opselect=C  inp2=PCIN>>17  opr=+  inp1=P  carry=CIN  dbl_ovrd=off  block_type=constant
      settings: block_version=VER_STRING_GOES_HERE
  zero14 : xbsIndex_r4/Constant  const=0  gui_display_data_type=Fixed-point  arith_type=Unsigned  n_bits=2  bin_pt=0  preci_type=Single  exp_width=8  frac_width=24  explicit_period=off  period=1  equ=P=C  opselect=C  inp2=PCIN>>17  opr=+  inp1=P  carry=CIN  dbl_ovrd=off  block_type=constant
      settings: block_version=VER_STRING_GOES_HERE
  zero15 : xbsIndex_r4/Constant  const=0  gui_display_data_type=Fixed-point  arith_type=Unsigned  n_bits=4  bin_pt=0  preci_type=Single  exp_width=8  frac_width=24  explicit_period=off  period=1  equ=P=C  opselect=C  inp2=PCIN>>17  opr=+  inp1=P  carry=CIN  dbl_ovrd=off  block_type=constant
      settings: block_version=VER_STRING_GOES_HERE
  zero16 : xbsIndex_r4/Constant  const=0  gui_display_data_type=Fixed-point  arith_type=Unsigned  n_bits=4  bin_pt=0  preci_type=Single  exp_width=8  frac_width=24  explicit_period=off  period=1  equ=P=C  opselect=C  inp2=PCIN>>17  opr=+  inp1=P  carry=CIN  dbl_ovrd=off  block_type=constant
      settings: block_version=VER_STRING_GOES_HERE
  zero18 : xbsIndex_r4/Constant  const=0  gui_display_data_type=Fixed-point  arith_type=Unsigned  n_bits=15  bin_pt=0  preci_type=Single  exp_width=8  frac_width=24  explicit_period=off  period=1  equ=P=C  opselect=C  inp2=PCIN>>17  opr=+  inp1=P  carry=CIN  dbl_ovrd=off  block_type=constant
      settings: block_version=VER_STRING_GOES_HERE
  zero23 : xbsIndex_r4/Constant  const=0  gui_display_data_type=Fixed-point  arith_type=Unsigned  n_bits=2  bin_pt=0  preci_type=Single  exp_width=8  frac_width=24  explicit_period=off  period=1  equ=P=C  opselect=C  inp2=PCIN>>17  opr=+  inp1=P  carry=CIN  dbl_ovrd=off  block_type=constant
      settings: block_version=VER_STRING_GOES_HERE
  zero26 : xbsIndex_r4/Constant  const=0  gui_display_data_type=Fixed-point  arith_type=Unsigned  n_bits=31  bin_pt=0  preci_type=Single  exp_width=8  frac_width=24  explicit_period=off  period=1  equ=P=C  opselect=C  inp2=PCIN>>17  opr=+  inp1=P  carry=CIN  dbl_ovrd=off  block_type=constant
      settings: block_version=VER_STRING_GOES_HERE
  zero5 : xbsIndex_r4/Constant  const=NumSamps_Tx_IQ  gui_display_data_type=Fixed-point  arith_type=Unsigned  n_bits=16  bin_pt=0  preci_type=Single  exp_width=8  frac_width=24  explicit_period=on  period=1  equ=P=C  opselect=C  inp2=PCIN>>17  opr=+  inp1=P  carry=CIN  dbl_ovrd=off  block_type=constant
      settings: block_version=VER_STRING_GOES_HERE
  zero6 : xbsIndex_r4/Constant  const=NumSamps_Rx_IQ  gui_display_data_type=Fixed-point  arith_type=Unsigned  n_bits=16  bin_pt=0  preci_type=Single  exp_width=8  frac_width=24  explicit_period=on  period=1  equ=P=C  opselect=C  inp2=PCIN>>17  opr=+  inp1=P  carry=CIN  dbl_ovrd=off  block_type=constant
      settings: block_version=VER_STRING_GOES_HERE
  tag scope: RFA_BUFFER_SEL=global, RFA_RX_BUF_EN=global, RFA_RX_COUNTER_RESET=global, RFA_TX_BUF_EN=global, RFA_TX_COUNTER_RESET=global, RFB_BUFFER_SEL=global, RFB_RX_BUF_EN=global, RFB_RX_COUNTER_RESET=global, RFB_TX_BUF_EN=global, RFB_TX_COUNTER_RESET=global, RFC_BUFFER_SEL=global, RFC_RX_BUF_EN=global, RFC_RX_COUNTER_RESET=global, RFC_TX_BUF_EN=global, RFC_TX_COUNTER_RESET=global, RFD_BUFFER_SEL=global, RFD_RX_BUF_EN=global, RFD_RX_COUNTER_RESET=global, RFD_TX_BUF_EN=global, RFD_TX_COUNTER_RESET=global, RF_RX_IQ_BUF_RD_BYTE_OFFSET=global, RF_RX_IQ_BUF_WR_BYTE_OFFSET=global, RF_RX_IQ_RSSI_ERROR_CLR=global, RF_RX_IQ_THRESHOLD=global, RF_TX_IQ_BUF_WR_BYTE_OFFSET=global, RF_TX_IQ_ERROR_CLR=global, RF_TX_IQ_THRESHOLD=global, RX_LENGTH=global, TX_DELAY=global, TX_LENGTH=global
  wires:
  TxDelay/1 -> [TX_DELAY]
  [AGC_Done_Detect] -> AGCDoneAddr/2, Radio1AGCDoneRSSI/2, Radio3AGCDoneRSSI/2
  Convert4/1 -> AGCDoneAddr/1
  Concat3/1 -> Radio3AGCDoneRSSI/1
  Concat2/1 -> Radio1AGCDoneRSSI/1
  From Register16/1 -> RFx Sel/1(32b)
  RFx Sel/1(A) -> [RFA_RX_BUF_EN]
  RFx Sel/2(B) -> [RFB_RX_BUF_EN]
  RFx Sel/3(C) -> [RFC_RX_BUF_EN]
  RFx Sel/4(D) -> [RFD_RX_BUF_EN]
  From Register1/1 -> RFx Sel2/1(32b)
  RFx Sel2/1(A) -> [RFA_TX_BUF_EN]
  RFx Sel2/2(B) -> [RFB_TX_BUF_EN]
  RFx Sel2/3(C) -> [RFC_TX_BUF_EN]
  RFx Sel2/4(D) -> [RFD_TX_BUF_EN]
  AGCDoneAddr/1 -> Terminator/1
  Radio1AGCDoneRSSI/1 -> Terminator1/1
  Radio3AGCDoneRSSI/1 -> Terminator3/1
  zero2/1 -> To Register1/2
  To Register1/1 -> Terminator6/1
  DESIGN_VER/1 -> Register/1
  zero3/1 -> To Register2/2
  Register/1 -> To Register2/1
  zero4/1 -> To Register3/2
  Concat1/1 -> To Register3/1
  zero5/1 -> Concat1/1
  zero6/1 -> Concat1/2
  To Register3/1 -> Terminator7/1
  To Register2/1 -> Terminator8/1
  From Register5/1 -> [TX_LENGTH]
  [WR_ADDR] -> Convert4/1
  From Register6/1 -> [RX_LENGTH]
  From Register13/1 -> Config Bits/1(D)
  zero1/1 -> Concat2/3
  [RFA_RSSI] -> Concat2/4
  [RFB_RSSI] -> Concat2/2
  zero8/1 -> Concat2/1
  zero7/1 -> Concat3/3
  [RFC_RSSI] -> Concat3/4
  zero9/1 -> Concat3/1
  [RFD_RSSI] -> Concat3/2
  b[1:0]/1 -> [RFA_BUFFER_SEL]
  b[9:8]/1 -> [RFB_BUFFER_SEL]
  b[17:16]/1 -> [RFC_BUFFER_SEL]
  b[25:24]/1 -> [RFD_BUFFER_SEL]
  From Register2/1 -> b[1:0]/1, b[9:8]/1, b[17:16]/1, b[25:24]/1
  From Register7/1 -> [RF_RX_IQ_THRESHOLD]
  From Register9/1 -> [RF_RX_IQ_BUF_RD_BYTE_OFFSET]
  Concat4/1 -> To Register4/1
  zero10/1 -> To Register4/2
  [RF_RX_IQ_BUF_WR_BYTE_OFFSET_UPDATE] -> To Register5/1
  To Register4/1 -> Terminator2/1
  From Register4/1 -> [RF_RX_IQ_BUF_WR_BYTE_OFFSET]
  To Register5/1 -> Terminator4/1
  zero12/1 -> To Register5/2
  zero13/1 -> To Register6/2
  Concat5/1 -> To Register6/1
  To Register6/1 -> Terminator5/1
  [RF_RX_IQ_BUF_OCCUPANCY] -> Concat5/2
  zero14/1 -> Concat5/1
  Constant2/1 -> DESIGN_VER/1
  Concat6/1 -> To Register1/1
  RFA_G_RF/1 -> Delay4/1
  RFA_G_BB/1 -> Delay5/1
  Constant6/1 -> RFA_G_RF/1
  Constant7/1 -> RFA_G_BB/1
  RFB_G_RF/1 -> Delay1/1
  RFB_G_BB/1 -> Delay2/1
  Constant3/1 -> RFB_G_RF/1
  Constant4/1 -> RFB_G_BB/1
  RFC_G_RF/1 -> Delay3/1
  RFC_G_BB/1 -> Delay6/1
  Constant5/1 -> RFC_G_RF/1
  Constant8/1 -> RFC_G_BB/1
  RFD_G_RF/1 -> Delay7/1
  RFD_G_BB/1 -> Delay8/1
  Constant9/1 -> RFD_G_RF/1
  Constant10/1 -> RFD_G_BB/1
  [AGC_Done_Detect] -> To Register7/2
  To Register7/1 -> Terminator9/1
  Concat7/1 -> Register3/1
  Register3/1 -> Register2/1
  Register2/1 -> Register1/1
  Register1/1 -> Convert1/1
  Convert1/1 -> To Register7/1
  RFA_RXHP/1 -> Delay9/1
  Constant11/1 -> RFA_RXHP/1
  RFB_RXHP/1 -> Delay10/1
  Constant1/1 -> RFB_RXHP/1
  RFC_RXHP/1 -> Delay11/1
  Constant12/1 -> RFC_RXHP/1
  RFD_RXHP/1 -> Delay12/1
  Constant13/1 -> RFD_RXHP/1
  Concat10/1 -> Concat7/1
  Concat9/1 -> Concat7/2
  Concat8/1 -> Concat7/3
  Concat/1 -> Concat7/4
  Delay12/1 -> Concat10/1
  Delay7/1 -> Concat10/2
  Delay8/1 -> Concat10/3
  Delay11/1 -> Concat9/1
  Delay3/1 -> Concat9/2
  Delay6/1 -> Concat9/3
  Delay10/1 -> Concat8/1
  Delay1/1 -> Concat8/2
  Delay2/1 -> Concat8/3
  Delay9/1 -> Concat/1
  Delay4/1 -> Concat/2
  Delay5/1 -> Concat/3
  AGCDoneAddr1/1 -> Terminator10/1
  Constant14/1 -> DRAM_INIT_DONE/1
  zero18/1 -> Concat6/1
  DRAM_INIT_DONE/1 -> Concat6/2
  zero19/1 -> AGCDoneAddr1/2
  AGCDoneAddr2/1 -> Terminator11/1
  zero20/1 -> AGCDoneAddr2/2
  From Register10/1 -> Timer64/2(Load MSB)
  From Register8/1 -> Timer64/3(Load LSB)
  Timer64/1(CNT_MSB) -> AGCDoneAddr2/1
  Timer64/2(CNT_LSB) -> AGCDoneAddr1/1
  [LOAD_TIMER_64] -> Timer64/1(Load)
  From Register14/1 -> [RF_TX_IQ_THRESHOLD]
  From Register11/1 -> [RF_TX_IQ_BUF_WR_BYTE_OFFSET]
  [RF_TX_IQ_BUF_RD_BYTE_OFFSET] -> To Register8/1
  To Register8/1 -> Terminator12/1
  zero21/1 -> To Register8/2
  zero22/1 -> To Register9/2
  Concat11/1 -> To Register9/1
  To Register9/1 -> Terminator13/1
  [RF_TX_IQ_BUF_OCCUPANCY] -> Concat11/2
  zero23/1 -> Concat11/1
  b[0]/1 -> [RF_RX_IQ_RSSI_ERROR_CLR]
  b[8]/1 -> [RF_TX_IQ_ERROR_CLR]
  From Register12/1 -> b[0]/1, b[8]/1
  zero11/1 -> Concat4/4
  [RF_TX_IQ_INT] -> Concat4/5
  [RF_RX_IQ_RSSI_INT] -> Concat4/6
  zero24/1 -> Concat4/1
  [RF_TX_IQ_ERROR] -> Concat4/2
  [RF_RX_IQ_RSSI_ERROR] -> Concat4/3
  zero25/1 -> To Register10/2
  Concat12/1 -> To Register10/1
  To Register10/1 -> Terminator14/1
  [TX_TMP_BUF_WR_DONE] -> Concat12/2
  zero26/1 -> Concat12/1
  zero16/1 -> Concat6/3
  Concat13/1 -> Concat6/4
  zero15/1 -> Concat6/5
  Concat14/1 -> Concat6/6
  zero17/1 -> To Register11/2
  RFA Tx Counter/1 -> To Register11/1
  To Register11/1 -> Terminator15/1
  zero27/1 -> To Register12/2
  RFB Tx Counter/1 -> To Register12/1
  To Register12/1 -> Terminator16/1
  zero28/1 -> To Register13/2
  RFC Tx Counter/1 -> To Register13/1
  To Register13/1 -> Terminator17/1
  zero29/1 -> To Register14/2
  RFD Tx Counter/1 -> To Register14/1
  To Register14/1 -> Terminator18/1
  zero30/1 -> To Register15/2
  RFA Rx Counter/1 -> To Register15/1
  To Register15/1 -> Terminator19/1
  zero31/1 -> To Register16/2
  RFB Rx Counter/1 -> To Register16/1
  To Register16/1 -> Terminator20/1
  zero32/1 -> To Register17/2
  RFC Rx Counter/1 -> To Register17/1
  To Register17/1 -> Terminator21/1
  zero33/1 -> To Register18/2
  RFD Rx Counter/1 -> To Register18/1
  To Register18/1 -> Terminator22/1
  COUNTER_RESET/1(RFA_TX) -> [RFA_TX_COUNTER_RESET]
  COUNTER_RESET/2(RFB_TX) -> [RFB_TX_COUNTER_RESET]
  COUNTER_RESET/3(RFC_TX) -> [RFC_TX_COUNTER_RESET]
  COUNTER_RESET/4(RFD_TX) -> [RFD_TX_COUNTER_RESET]
  COUNTER_RESET/5(RFA_RX) -> [RFA_RX_COUNTER_RESET]
  COUNTER_RESET/6(RFB_RX) -> [RFB_RX_COUNTER_RESET]
  COUNTER_RESET/7(RFC_RX) -> [RFC_RX_COUNTER_RESET]
  COUNTER_RESET/8(RFD_RX) -> [RFD_RX_COUNTER_RESET]
  From Register3/1 -> COUNTER_RESET/1(32b)
  [RFA_TX_COUNTER_RESET] -> RFA Tx Counter/1
  Posedge/1(Q) -> RFA Tx Counter/2
  [RFB_TX_COUNTER_RESET] -> RFB Tx Counter/1
  Posedge1/1(Q) -> RFB Tx Counter/2
  [RFC_TX_COUNTER_RESET] -> RFC Tx Counter/1
  Posedge2/1(Q) -> RFC Tx Counter/2
  [RFD_TX_COUNTER_RESET] -> RFD Tx Counter/1
  Posedge3/1(Q) -> RFD Tx Counter/2
  [RFA_RX_COUNTER_RESET] -> RFA Rx Counter/1
  Posedge4/1(Q) -> RFA Rx Counter/2
  [RFB_RX_COUNTER_RESET] -> RFB Rx Counter/1
  Posedge5/1(Q) -> RFB Rx Counter/2
  [RFC_RX_COUNTER_RESET] -> RFC Rx Counter/1
  Posedge6/1(Q) -> RFC Rx Counter/2
  [RFD_RX_COUNTER_RESET] -> RFD Rx Counter/1
  Posedge7/1(Q) -> RFD Rx Counter/2
  RF RUNNING/1(RFA_TX) -> Posedge/1(D), Concat14/4
  RF RUNNING/2(RFB_TX) -> Posedge1/1(D), Concat14/3
  RF RUNNING/3(RFC_TX) -> Posedge2/1(D), Concat14/2
  RF RUNNING/4(RFD_TX) -> Posedge3/1(D), Concat14/1
  RF RUNNING/5(RFA_RX) -> Posedge4/1(D), Concat13/4
  RF RUNNING/6(RFB_RX) -> Posedge5/1(D), Concat13/3
  RF RUNNING/7(RFC_RX) -> Posedge6/1(D), Concat13/2
  RF RUNNING/8(RFD_RX) -> Posedge7/1(D), Concat13/1

== system w3_warplab_buffers/Posedge 0 ==
  D : Inport
  Delay : xbsIndex_r4/Delay  rst=off  infoeditControl=Selection of Reset will increase slice count due to use of real FFs and instead of SRLs  en=off  latency=1  dbl_ovrd=off  reg_retiming=off  block_type=delay
      settings: infoedit=Hardware notes: A delay line is a chain, each link of which is an SRL16 followed by a flip-flop. If register retiming is enabled, the delay line is a chain of flip-flops.  block_version=8.2
  Inverter : xbsIndex_r4/Inverter  en=off  latency=0  dbl_ovrd=off  block_type=inv
      settings: block_version=8.2
  Logical : xbsIndex_r4/Logical  logical_function=AND  inputs=2  en=off  latency=0  precision=Full  arith_type=Unsigned  n_bits=16  bin_pt=0  align_bp=on  dbl_ovrd=off  block_type=logical
      settings: block_version=8.2
  Q : Outport
  wires:
  Logical/1 -> Q/1
  Delay/1 -> Logical/2
  Inverter/1 -> Delay/1
  D/1 -> Logical/1, Inverter/1

== system w3_warplab_buffers/Posedge 1 ==
  D : Inport
  Delay : xbsIndex_r4/Delay  rst=off  infoeditControl=Selection of Reset will increase slice count due to use of real FFs and instead of SRLs  en=off  latency=1  dbl_ovrd=off  reg_retiming=off  block_type=delay
      settings: infoedit=Hardware notes: A delay line is a chain, each link of which is an SRL16 followed by a flip-flop. If register retiming is enabled, the delay line is a chain of flip-flops.  block_version=8.2
  Inverter : xbsIndex_r4/Inverter  en=off  latency=0  dbl_ovrd=off  block_type=inv
      settings: block_version=8.2
  Logical : xbsIndex_r4/Logical  logical_function=AND  inputs=2  en=off  latency=0  precision=Full  arith_type=Unsigned  n_bits=16  bin_pt=0  align_bp=on  dbl_ovrd=off  block_type=logical
      settings: block_version=8.2
  Q : Outport
  wires:
  D/1 -> Inverter/1, Logical/1
  Inverter/1 -> Delay/1
  Delay/1 -> Logical/2
  Logical/1 -> Q/1

== system w3_warplab_buffers/RFA Rx Buffers ==
  RSSI : Inport
  I/Q : Inport  Port=2
  Addr : Inport  Port=3
  WE : Inport  Port=4
  EN : Inport  Port=5
  Convert1 : xbsIndex_r4/Convert  gui_display_data_type=Fixed-point  arith_type=Boolean  n_bits=16  bin_pt=14  float_type=Single  exp_bits=8  fraction_bits=24  quantization=Truncate  overflow=Wrap  en=off  latency=0  dbl_ovrd=off  pipeline=off  block_type=convert
      settings: block_version=8.2
  Gateway Out : xbsIndex_r4/Gateway Out  inherit_from_input=off  hdl_port=off  timing_constraint=None  locs_specified=off  LOCs={}  UseAsDAC=off  DACChannel='1'  block_type=gatewayout
      settings: infoedit="Gateway out block.  Converts Xilinx fixed point inputs into ouputs of type Simulink integer, double, or fixed point.<P><P>Hardware notes:  In hardware these blocks become top level output ports or are discarded, depending on how they are configured."  block_version=10.1.2
  Gateway Out1 : xbsIndex_r4/Gateway Out  inherit_from_input=off  hdl_port=off  timing_constraint=None  locs_specified=off  LOCs={}  UseAsDAC=off  DACChannel='1'  block_type=gatewayout
      settings: infoedit="Gateway out block.  Converts Xilinx fixed point inputs into ouputs of type Simulink integer, double, or fixed point.<P><P>Hardware notes:  In hardware these blocks become top level output ports or are discarded, depending on how they are configured."  block_version=10.1.2
  I/Q Buffer : Subsystem
  Logical : xbsIndex_r4/Logical  logical_function=AND  inputs=2  en=off  latency=0  precision=Full  arith_type=Unsigned  n_bits=16  bin_pt=0  align_bp=on  dbl_ovrd=off  block_type=logical
      settings: block_version=9.1.01
  RSSI Buffer : Subsystem
  Scope : Scope  NumInputPorts=2
      settings: YMin=-5~-5  YMax=5~5  SaveName=ScopeData2  MaxDataPoints=40000
  wires:
  Logical/1 -> Gateway Out1/1, I/Q Buffer/3(WE), RSSI Buffer/3(WE)
  Addr/1 -> Gateway Out/1, I/Q Buffer/1(Addr), RSSI Buffer/1(Addr)
  WE/1 -> Logical/1
  EN/1 -> Convert1/1
  Convert1/1 -> Logical/2
  I/Q/1 -> I/Q Buffer/2(I/Q_32b)
  Gateway Out/1 -> Scope/1
  Gateway Out1/1 -> Scope/2
  RSSI/1 -> RSSI Buffer/2(RSSI)
